simulink model "ACC_TESTE_2026_pid"  (R2026a)
settings: Solver=VariableStepAuto  StopTime=70.0
values from neighbouring files (symbols this model uses):
  D0 = 150    [INIT_ACC_2026.m]
  Vf0 = 18    [INIT_ACC_2026.m]
settings Model: Creator=ADM

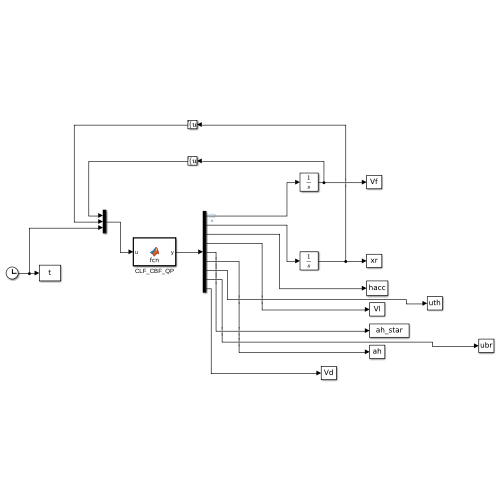
[thumbnail: Simulink's stored preview of the top-level diagram]
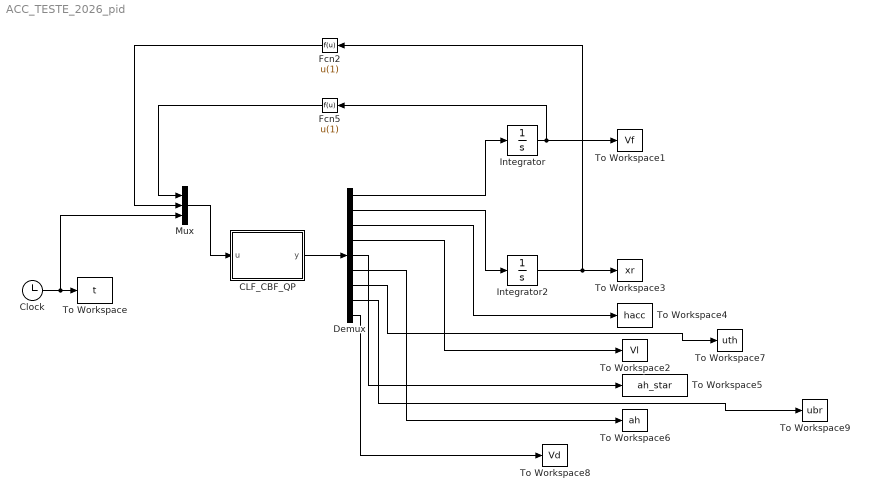
== system ACC_TESTE_2026_pid ==
  CLF_CBF_QP : MATLAB Function  TreatAsAtomicUnit=on
  Clock : Clock
  Demux : Demux  Outputs=9
  Fcn2 : Fcn  Expr=u(1)
  Fcn5 : Fcn  Expr=u(1)
  Integrator : Integrator  InitialCondition=Vf0
  Integrator2 : Integrator  InitialCondition=D0
  Mux : Mux  Inputs=3
  To Workspace : ToWorkspace  VariableName=t  SampleTime=0.02
  To Workspace1 : ToWorkspace  VariableName=Vf  SampleTime=-1
  To Workspace2 : ToWorkspace  VariableName=Vl  SampleTime=-1
  To Workspace3 : ToWorkspace  VariableName=xr  SampleTime=-1
  To Workspace4 : ToWorkspace  VariableName=hacc  SampleTime=-1
  To Workspace5 : ToWorkspace  VariableName=ah_star  SampleTime=-1
  To Workspace6 : ToWorkspace  VariableName=ah  SampleTime=-1
  To Workspace7 : ToWorkspace  VariableName=uth  SampleTime=-1
  To Workspace8 : ToWorkspace  VariableName=Vd  SampleTime=-1
  To Workspace9 : ToWorkspace  VariableName=ubr  SampleTime=-1
  wires:
  CLF_CBF_QP/1(y) -> Demux/1
  Clock/1 -> Mux/3, To Workspace/1
  Integrator2/1 -> To Workspace3/1, Fcn2/1
  Demux/1 -> Integrator/1
  Demux/4 -> To Workspace2/1
  Fcn2/1 -> Mux/2
  Demux/2 -> Integrator2/1
  Mux/1 -> CLF_CBF_QP/1(u)
  Integrator/1 -> To Workspace1/1, Fcn5/1
  Demux/3 -> To Workspace4/1
  Fcn5/1 -> Mux/1
  Demux/5 -> To Workspace5/1
  Demux/6 -> To Workspace6/1
  Demux/9 -> To Workspace8/1
  Demux/7 -> To Workspace7/1
  Demux/8 -> To Workspace9/1

== matlab function ACC_TESTE_2026_pid/CLF_CBF_QP ==
  settings: updateMethod=DISCRETE
  data: u input; y output
function y = fcn(u)
% ============================================================
% ACC — Arquitetura de Dois Níveis (Chinelato et al., 2023)
% Nível Superior: CLF-CBF-QP (u = aceleração, convenção Chinelato)
% Nível Inferior: PID simplificado (throttle/freio), SEM atraso
%                 de atuador — o PID atua diretamente, usando
%                 `persistent` para manter memória (termo integral)
%                 sem precisar de blocos extras no Simulink.
% ============================================================

% Estados
Vf = u(1);
xr = u(2);
% Tempo
t  = u(3);

% --- Parâmetros do veículo ---
m  = 1650;
f0 = 0.1;
f1 = 5;
f2 = 0.25;

% --- Perfil do veículo líder (idêntico aos arquivos anteriores) ---
if(t <= 10)
    Vl = 10;
elseif(t>10 && t<=20)
    Vl = -2+1.2*t;
elseif(t>20 && t<=30)
    Vl = 22;
elseif(t>30 && t<=40)
    Vl = 7+0.5*t;
elseif(t>40 && t<=50)
    Vl = 27;
elseif(t>50 && t<=60)
    Vl = 77-t;
else
    Vl = 17;
end

Fr = f0 + f1*Vf + f2*Vf*Vf;

% ============================================================
% NÍVEL SUPERIOR — CLF-CBF-QP (Chinelato et al., 2023, Seção 4)
% Convenção: uacc = Fw/Mh (aceleração, NÃO força) => g_acc=[1;0]
% ============================================================
Vd      = 22;     % velocidade de cruzeiro desejada
tau_th  = 1.8;     % time headway (≡ Td)
cVacc   = 10;      % taxa de convergência da CLF (≡ c)
gammacc = 10;       % agressividade da CBF (≡ lambda), mudei de 1 para 10
pdacc   = 10;      % peso da folga — validado empiricamente (ver simulacao.md)

Vacc = (Vf-Vd)^2;
LfVacc = -2*(Vf-Vd)*Fr/m;
LgVacc = 2*(Vf-Vd);

hacc = xr - tau_th*Vf;
Lfhacc = Vl - Vf + tau_th*Fr/m;
Lghacc = -tau_th;

% Custo (Chinelato, eq. 33): Hacc SEM 1/m^2 — aqui u já é aceleração
Hacc = 2*[1 0; 0 pdacc];
Facc = -2*[Fr/m; 0];

A = [LgVacc -1; -Lghacc 0];
b = [-LfVacc-cVacc*Vacc; Lfhacc+gammacc*hacc];

ucont = [0;0];
coder.extrinsic('QPhild');
ucont = QPhild(Hacc,Facc,A,b);
uacc_star = ucont(1,1);        % demanda de atuação TOTAL (antes do arrasto)
ah_star   = uacc_star - Fr/m;  % a_h*  — aceleração desejada, líquida (para o nível inferior)

% ============================================================
% NÍVEL INFERIOR — PID simplificado (throttle + freio)
% Sem dinâmica de atuador: o "erro" só aparece quando a demanda
% de aceleração satura a capacidade máxima de throttle/freio.
% ============================================================
persistent int_eth int_ebr ah_ant
if isempty(int_eth)
    int_eth = 0; int_ebr = 0; ah_ant = 0;
end

% Capacidades máximas dos atuadores (aceleração líquida, m/s^2)
a_th_max = 3.0;   % aceleração máxima via acelerador
a_br_max = 6.0;   % desaceleração máxima via freio

% Ganhos do PID (throttle e freio, sintonizados empiricamente)
Kp_th = 0.6;  Ki_th = 0.05;  Kd_th = 0.02;
Kp_br = 0.6;  Ki_br = 0.05;  Kd_br = 0.02;

% Erros (Chinelato, eq. 36-37): eth = ah - a*h ; ebr = a*h - ah
% Usa ah do passo anterior (persistent) — implementação discreta padrão
eth = ah_ant - ah_star;
ebr = ah_star - ah_ant;

Ts = 0.02; % período de amostragem aproximado (ajuste conforme o solver)
int_eth = int_eth + eth*Ts;
int_ebr = int_ebr + ebr*Ts;

uth_cmd = Kp_th*(-eth) + Ki_th*(-int_eth); % ação corretiva do throttle
ubr_cmd = Kp_br*(-ebr) + Ki_br*(-int_ebr); % ação corretiva do freio

% Mapeamento inicial (proporcional) + correção do PID, saturado em [0,100]%
if ah_star >= 0
    uth = min(100, max(0, 100*ah_star/a_th_max + uth_cmd));
    ubr = 0;
else
    uth = 0;
    ubr = min(100, max(0, 100*(-ah_star)/a_br_max + ubr_cmd));
end

% Aceleração REAL entregue pelos atuadores (o que o nível inferior
% de fato consegue produzir — pode saturar e não bater com ah_star)
ah = (uth/100)*a_th_max - (ubr/100)*a_br_max;
ah_ant = ah; % memória para o próximo passo

% ============================================================
% Dinâmica do veículo — usa ah REAL (não ah_star!) — é isso que
% torna a arquitetura de dois níveis genuína: o que o carro faz
% de fato passa pelo filtro do nível inferior.
% ============================================================
xponto = [ah - Fr/m + Fr/m; Vl - Vf]; % dVf/dt = ah  (ah já é líquido)
% (equivalente a xponto(1) = ah, mantido explícito por clareza)
xponto(1) = ah;

y = [xponto(1,1); xponto(2,1); hacc; Vl; ah_star; ah; uth; ubr; Vd];
